simulink subsystem "plant"  (R2026a)
settings: Solver=VariableStepAuto
settings Model: DataDictionary=plantParams.sldd  EnableAccessToBaseWorkspace=off  Creator=maxhu  LastModifiedBy=maxhu

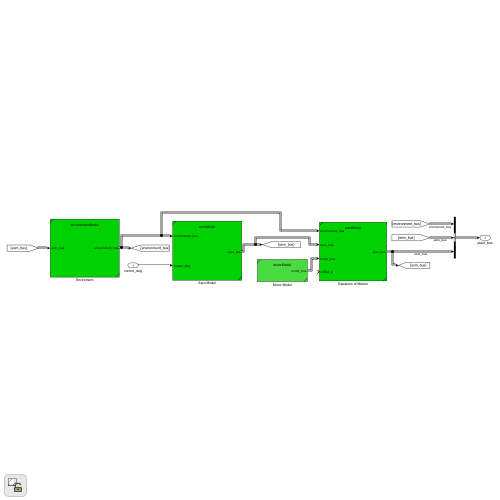
[thumbnail: Simulink's stored preview of the top-level diagram]
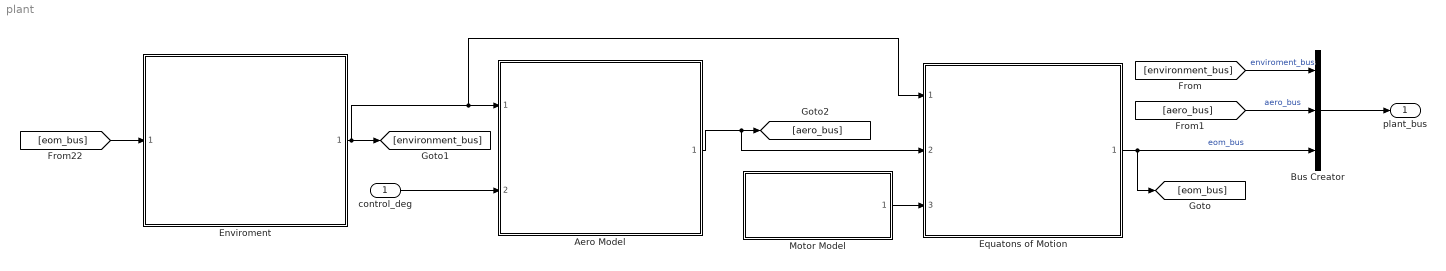
== system plant ==
  control_deg : Inport
  Aero Model : Subsystem  ReferencedSubsystem=aeroModel
      settings: PermitHierarchicalResolution=None
  Bus Creator : BusCreator  Inputs=3
  Enviroment : Subsystem  ReferencedSubsystem=environmentModel
      settings: PermitHierarchicalResolution=None
  Equatons of Motion : Subsystem  ReferencedSubsystem=eomModel
      settings: PermitHierarchicalResolution=None
  Motor Model : Subsystem  ReferencedSubsystem=motorModel
  plant_bus : Outport
  wires:
  Enviroment/1 -> Equatons of Motion/1, Aero Model/1, [environment_bus]
  [eom_bus] -> Enviroment/1
  Aero Model/1 -> Equatons of Motion/2, [aero_bus]
  [environment_bus] -> Bus Creator/1  "enviroment_bus"
  control_deg/1 -> Aero Model/2
  Equatons of Motion/1 -> Bus Creator/3, [eom_bus]  "eom_bus"
  [aero_bus] -> Bus Creator/2  "aero_bus"
  Bus Creator/1 -> plant_bus/1
  Motor Model/1 -> Equatons of Motion/3
